simulink library "rw_torque_allocation_lib"  (R2018b)
settings: Solver=VariableStepAuto  StartTime=0.0  StopTime=10.0  RelTol=1e-3
undefined symbols (not defined in the file or in its folder): fsw_params
settings Model: Creator=Taylor  LastModifiedBy=Taylor

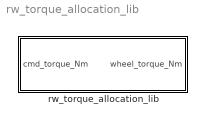
== system rw_torque_allocation_lib ==
  rw_torque_allocation_lib : Subsystem

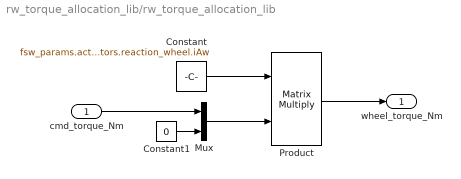
== system rw_torque_allocation_lib/rw_torque_allocation_lib ==
  cmd_torque_Nm : Inport
  Constant : Constant  Value=fsw_params.actuators.reaction_wheel.iAw
  Constant1 : Constant  Value=0
  Mux : Mux  Inputs=[3 1]
  Product : Product  Multiplication=Matrix(*)
  wheel_torque_Nm : Outport
  wires:
  cmd_torque_Nm/1 -> Mux/1
  Constant/1 -> Product/1
  Constant1/1 -> Mux/2
  Mux/1 -> Product/2
  Product/1 -> wheel_torque_Nm/1
